simulink model "Feedforward_ROS"  (R2022b)
settings: Solver=FixedStepAuto  StartTime=0.0  StopTime=45  FixedStep=0.02  MaxStep=0.1  RelTol=1e-3
undefined symbols (not defined in the file): unicycle, X, Y
libraries: robotlib x3, simulink_extras x2
settings Model: Creator=hp 2021  LastModifiedBy=mustacchim
settings OptimizationCC: EnhancedBackFolding=on  PassReuseOutputArgsAs=Individual arguments  ZeroExternalMemoryAtStartup=off  ZeroInternalMemoryAtStartup=off  MaxStackSize=64  OptimizeBlockOrder=speed  DifferentSizesBufferReuse=on  OptimizationCustomize=off  EfficientTunableParamExpr=on
settings DebuggingCC: ParameterTunabilityLossMsg=error
settings HardwareCC: ProdBitPerPointer=32  ProdBitPerSizeT=32  ProdBitPerPtrDiffT=32  ProdLargestAtomicFloat=None  ProdIntDivRoundTo=Undefined  ProdEndianess=Unspecified  ProdWordSize=32  ProdHWDeviceType=Generic->Unspecified (assume 32-bit Generic)  UseEmbeddedCoderFeatures=off
settings ModelReferenceCC: EnableRefExpFcnMdlSchedulingChecks=on
settings SFSimCC: MATLABDynamicMemAlloc=off
settings RTWCC: Description=Embedded Coder  SystemTargetFile=ert.tlc  HardwareBoard=Robot Operating System (ROS)  TLCOptions="-aInlineSetEventsForThisBaseRateFcn=TLC_FALSE -aSuppressMultiTaskScheduler=TLC_FALSE  -aRateBasedStepFcn=0"  TemplateMakefile=ert_default_tmf  Toolchain=Catkin  TargetLang=C++
settings CodeAppCC: ForceParamTrailComments=on  IgnoreCustomStorageClasses=off  OperatorAnnotations=on  SimulinkDataObjDesc=on  SFDataObjDesc=on  InsertBlockDesc=on
settings ERTTargetCC: SupportNonInlinedSFcns=on

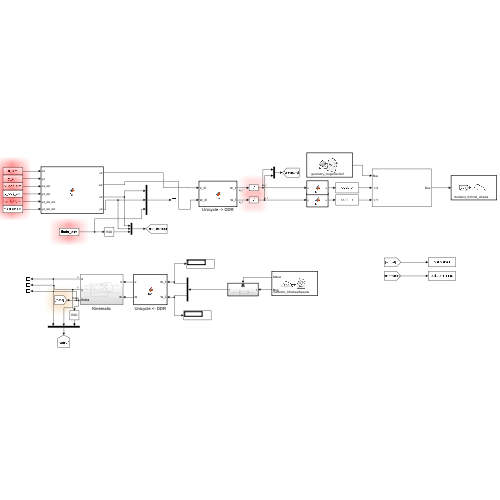
[thumbnail: Simulink's stored preview of the top-level diagram]
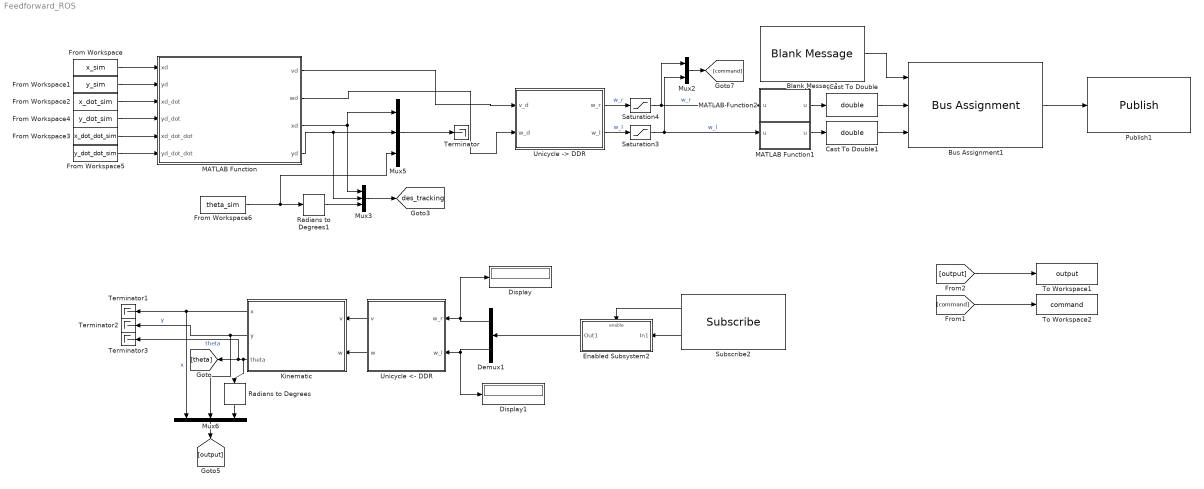
== system Feedforward_ROS ==
  Blank Message1 : robotlib/Blank Message  messageClass=Message  entityType=geometry_msgs/Vector3  messageType=geometry_msgs/Vector3  SampleTime=0.02  legacyBusStruct=off
      settings: LibrarySourceBlock=roslib/ROS/Blank Message
  Bus Assignment1 : BusAssignment  AssignedSignals=X,Y
  Cast To Double : DataTypeConversion  OutDataTypeStr=double  SaturateOnIntegerOverflow=off  RndMeth=Floor
  Cast To Double1 : DataTypeConversion  OutDataTypeStr=double  SaturateOnIntegerOverflow=off  RndMeth=Floor
  Demux1 : Demux  Outputs=2
  Display : Display
  Display1 : Display
  Enabled Subsystem2 : Subsystem  TreatAsAtomicUnit=on
  From Workspace : FromWorkspace  VariableName=x_sim
  From Workspace1 : FromWorkspace  VariableName=y_sim
  From Workspace2 : FromWorkspace  VariableName=x_dot_sim
  From Workspace3 : FromWorkspace  VariableName=x_dot_dot_sim
  From Workspace4 : FromWorkspace  VariableName=y_dot_sim
  From Workspace5 : FromWorkspace  VariableName=y_dot_dot_sim
  From Workspace6 : FromWorkspace  VariableName=theta_sim
  Kinematic : Subsystem
  MATLAB Function : MATLAB Function  TreatAsAtomicUnit=on
  MATLAB Function1 : MATLAB Function  TreatAsAtomicUnit=on
  MATLAB Function2 : MATLAB Function  TreatAsAtomicUnit=on
  Mux2 : Mux  Inputs=2
  Mux3 : Mux  Inputs=3
  Mux5 : Mux  Inputs=3
  Mux6 : Mux  Inputs=3
  Publish1 : robotlib/Publish  topicSource=Select from ROS network  topic=/turtlebot_03/cmd_wheels  messageType=geometry_msgs/Vector3  legacyBusStruct=off  messageQueueLength=1
      settings: LibrarySourceBlock=roslib/ROS/Publish
  Radians to Degrees : simulink_extras/Transformations/Radians to Degrees
  Radians to Degrees1 : simulink_extras/Transformations/Radians to Degrees
  Saturation3 : Saturate  UpperLimit=unicycle.omegaWheelMax  LowerLimit=unicycle.omegaWheelMin
  Saturation4 : Saturate  UpperLimit=unicycle.omegaWheelMax  LowerLimit=unicycle.omegaWheelMin
  Subscribe2 : robotlib/Subscribe  topicSource=Select from ROS network  topic=/turtlebot_03/wheelSpeeds  messageType=geometry_msgs/Vector3  SampleTime=0.02  legacyBusStruct=off  messageQueueLength=1
      settings: LibrarySourceBlock=roslib/ROS/Subscribe
  Terminator{,1..3} (4 alike) : Terminator
  To Workspace1 : ToWorkspace  VariableName=output  SaveFormat=Structure With Time  SampleTime=-1
  To Workspace2 : ToWorkspace  VariableName=command  SaveFormat=Structure With Time  SampleTime=-1
  "Unicycle -> DDR" : MATLAB Function  TreatAsAtomicUnit=on
  Unicycle <- DDR : MATLAB Function  TreatAsAtomicUnit=on
  tag scope: des_tracking=global
  wires:
  [output] -> To Workspace1/1
  Blank Message1/1 -> Bus Assignment1/1
  "Unicycle -> DDR"/2(w_l) -> Saturation3/1  "w_l"
  Mux2/1 -> [command]
  Bus Assignment1/1 -> Publish1/1
  Saturation3/1 -> MATLAB Function1/1("u "), Mux2/2  "w_l"
  Saturation4/1 -> MATLAB Function2/1("u "), Mux2/1  "w_r"
  "Unicycle -> DDR"/1(w_r) -> Saturation4/1  "w_r"
  Cast To Double/1 -> Bus Assignment1/2
  Cast To Double1/1 -> Bus Assignment1/3
  MATLAB Function/3(xd) -> Mux5/1, Mux3/1
  Mux5/1 -> Terminator/1
  Radians to Degrees1/1 -> Mux3/3
  From Workspace2/1 -> MATLAB Function/3(xd_dot)
  From Workspace3/1 -> MATLAB Function/5(xd_dot_dot)
  From Workspace/1 -> MATLAB Function/1("xd ")
  Mux3/1 -> [des_tracking]
  From Workspace5/1 -> MATLAB Function/6(yd_dot_dot)
  From Workspace6/1 -> Radians to Degrees1/1, Mux5/3
  From Workspace1/1 -> MATLAB Function/2("yd ")
  From Workspace4/1 -> MATLAB Function/4(yd_dot)
  MATLAB Function/2(wd) -> "Unicycle -> DDR"/2(w_d)
  MATLAB Function/1(vd) -> "Unicycle -> DDR"/1(v_d)
  MATLAB Function/4(yd) -> Mux3/2, Mux5/2
  MATLAB Function1/1(u) -> Cast To Double1/1
  MATLAB Function2/1(u) -> Cast To Double/1
  Kinematic/1(x) -> Terminator1/1, Mux6/1  "x"
  Unicycle <- DDR/2(w) -> Kinematic/2(w)
  Radians to Degrees/1 -> Mux6/3
  Demux1/2 -> Display1/1, Unicycle <- DDR/2(w_l)
  Subscribe2/2 -> Enabled Subsystem2/1(In1)
  Kinematic/2(y) -> Terminator2/1, Mux6/2  "y"
  Demux1/1 -> Display/1, Unicycle <- DDR/1(w_r)
  Subscribe2/1 -> Enabled Subsystem2/Enable
  Kinematic/3(theta) -> Terminator3/1, [theta], Radians to Degrees/1  "theta"
  Unicycle <- DDR/1(v) -> Kinematic/1(v)
  Mux6/1 -> [output]
  Enabled Subsystem2/1(Out1) -> Demux1/1
  [command] -> To Workspace2/1

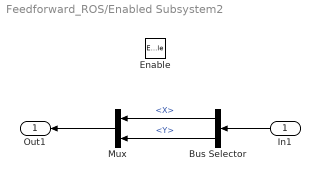
== system Feedforward_ROS/Enabled Subsystem2 ==
  In1 : Inport
  Enable : EnablePort
  Bus Selector : BusSelector  OutputSignals=X,Y
  Mux : Mux  Inputs=2
  Out1 : Outport
  wires:
  Mux/1 -> Out1/1
  Bus Selector/1 -> Mux/1  "<X>"
  Bus Selector/2 -> Mux/2  "<Y>"
  In1/1 -> Bus Selector/1

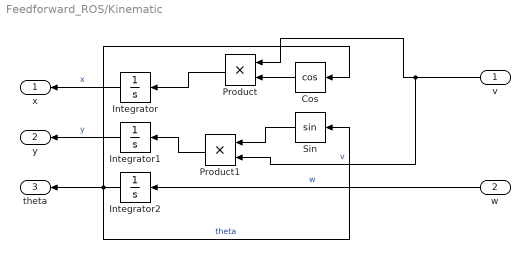
== system Feedforward_ROS/Kinematic ==
  v : Inport
  w : Inport  Port=2
  Cos : Trigonometry  Operator=cos
  Integrator : Integrator  InitialCondition=unicycle.ic.x
  Integrator1 : Integrator  InitialCondition=unicycle.ic.y
  Integrator2 : Integrator  InitialCondition=unicycle.ic.theta
  Product : Product
  Product1 : Product
  Sin : Trigonometry
  x : Outport
  y : Outport  Port=2
  theta : Outport  Port=3
  wires:
  w/1 -> Integrator2/1  "w"
  Product/1 -> Integrator/1
  v/1 -> Product/1, Product1/2  "v"
  Cos/1 -> Product/2
  Integrator1/1 -> y/1  "y"
  Integrator/1 -> x/1  "x"
  Integrator2/1 -> theta/1, Sin/1, Cos/1  "theta"
  Product1/1 -> Integrator1/1
  Sin/1 -> Product1/1

== matlab function Feedforward_ROS/MATLAB Function ==
  data: xd input; vd output; yd input; xd_dot input; yd_dot input; xd_dot_dot input; yd_dot_dot input; wd output; xd output; yd output
function [vd, wd, xd, yd] = fcn(xd, yd, xd_dot, yd_dot, xd_dot_dot, yd_dot_dot)
    
    vd = sqrt(xd_dot.^2 + yd_dot.^2);
    wd = (xd_dot.*yd_dot_dot - xd_dot_dot.*yd_dot) / (xd_dot.^2 + yd_dot.^2);

    xd = xd;
    yd = yd;

end

== matlab function Feedforward_ROS/MATLAB Function1 ==
  data: u input; u output
function u = fcn(u)


    if (isnan(u))
        u = 0.1;
    end

end

== matlab function Feedforward_ROS/MATLAB Function2 ==
  data: u input; u output
function u = fcn(u)

    if (isnan(u))
        u = 0.1;
    end

end

== matlab function Feedforward_ROS/Unicycle <- DDR ==
  data: w_r input; v output; w_l input; w output
function [v, w] = fcn(w_r, w_l)

    %#codegen
    coder.extrinsic('evalin')
    d = 0;                  % Needed in order to set variable class correctly
    r = 0;                  % Needed in order to set variable class correctly
    d = evalin('base','unicycle.d'); % Read value from workspace
    r = evalin('base','unicycle.r'); % Read value from workspace

    v = r*(w_r + w_l)/2; % rad/s
    w = r*(w_r - w_l)/d; % rad/s

end

== matlab function Feedforward_ROS/Unicycle -> DDR ==
  data: v_d input; w_r output; w_d input; w_l output
function [w_r, w_l] = fcn(v_d, w_d)

    %#codegen
    coder.extrinsic('evalin')
    d = 0;                  % Needed in order to set variable class correctly
    r = 0;                  % Needed in order to set variable class correctly
    d = evalin('base','unicycle.d'); % Read value from workspace
    r = evalin('base','unicycle.r'); % Read value from workspace

    w_r = ((2 * v_d) + (w_d * d)) / (2 * r);
    w_l = ((2 * v_d) - (w_d * d)) / (2 * r);

end
